simulink model "DecentralizedWindParkModel"  (Simulink 8.2)
settings: Solver=ode45  StartTime=0.0  StopTime=inf  RelTol=1e-3
undefined symbols (not defined in the file): Take, Turbine_Library, Turbine_Profile
libraries: DDSLibrary x4
settings Model: Creator=thomas  LastModifiedBy=thomas
settings DataIOCC: SignalLoggingSaveFormat=Dataset
settings OptimizationCC: ExpressionDepthLimit=128
settings DebuggingCC: FcnCallInpInsideContextMsg=EnableAllAsError  StateNameClashWarn=none
settings GRTTargetCC: CombineOutputUpdateFcns=on  GRTInterface=off

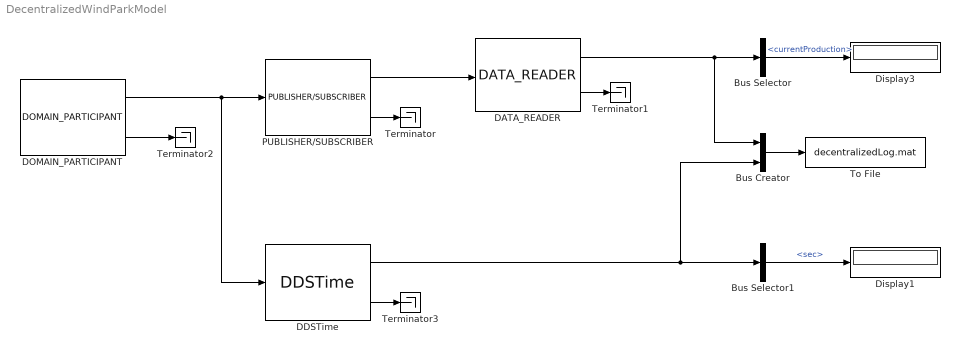
== system DecentralizedWindParkModel ==
  Bus Creator : BusCreator  Inputs=2
  Bus Selector : BusSelector  OutputSignals=currentProduction
  Bus Selector1 : BusSelector  OutputSignals=sec
  DATA_READER : DDSLibrary/DATA_READER  SFunctionSpec=)  SParam2=TurbineMessage  SParam3=Cluster 1  SParam4=-1  SParam1=on  SParam6=1  SParam7=Take()  SParam5=Turbine_Library::Turbine_Profile
  DDSTime : DDSLibrary/DDSTime  SFunctionSpec=[]
  DOMAIN_PARTICIPANT : DDSLibrary/DOMAIN_PARTICIPANT  SFunctionSpec=)  SParam1=-1  SParam2=Turbine_Library::Turbine_Profile  SParam3=0
  Display1 : Display
  Display3 : Display
  PUBLISHER/SUBSCRIBER : DDSLibrary/PUBLISHER//SUBSCRIBER  SFunctionSpec=)  SParam2=Subscriber  SParam1=-1  SParam3=Turbine_Library::Turbine_Profile
  Terminator{,1..3} (4 alike) : Terminator
  To File : ToFile  Filename=decentralizedLog.mat  MatrixName=decentralizedLog  SaveFormat=Timeseries
  wires:
  PUBLISHER/SUBSCRIBER/1 -> DATA_READER/1
  DATA_READER/1 -> Bus Creator/1, Bus Selector/1
  DATA_READER/2 -> Terminator1/1
  Bus Selector/1 -> Display3/1  "<currentProduction>"
  PUBLISHER/SUBSCRIBER/2 -> Terminator/1
  DOMAIN_PARTICIPANT/2 -> Terminator2/1
  Bus Selector1/1 -> Display1/1  "<sec>"
  DDSTime/2 -> Terminator3/1
  Bus Creator/1 -> To File/1
  DDSTime/1 -> Bus Creator/2, Bus Selector1/1
  DOMAIN_PARTICIPANT/1 -> DDSTime/1, PUBLISHER/SUBSCRIBER/1
